simulink model "optimized_area_multi_module_phase_shift_generator_built_in_counter"  (R2025b)
settings: Solver=FixedStepDiscrete  StartTime=0.0  StopTime=10e3  RelTol=1e-3
libraries: hdlsllib x1
settings Model: DataTypeOverride=Off  FPTShortcutValueString='{{},{''BaselineRun'',1,1,1,''BaselineRun'','''',{},''M'',''F'',''''}}'  Creator=KoayXianCong  LastModifiedBy=KoayXianCong
settings OptimizationCC: BlockReduction=off  ConditionallyExecuteInputs=off  DefaultParameterBehavior=Inlined  InheritOutputTypeSmallerThanSingle=on
settings DebuggingCC: SignalRangeChecking=warning  ArtificialAlgebraicLoopMsg=error  SingleTaskRateTransMsg=error
settings HardwareCC: ProdBitPerPointer=32.0  ProdBitPerSizeT=32.0  ProdBitPerPtrDiffT=32.0  ProdLargestAtomicFloat=None  ProdIntDivRoundTo=Undefined  ProdEndianess=Unspecified  ProdWordSize=32.0  ProdHWDeviceType=ASIC/FPGA->ASIC/FPGA  TargetBitPerPointer=64.0  TargetBitPerSizeT=64.0  TargetBitPerPtrDiffT=64.0  TargetLongLongMode=on  TargetIntDivRoundTo=Zero  TargetEndianess=LittleEndian  TargetWordSize=64.0  TargetHWDeviceType=Custom Processor->MATLAB Host Computer  ProdEqTarget=off

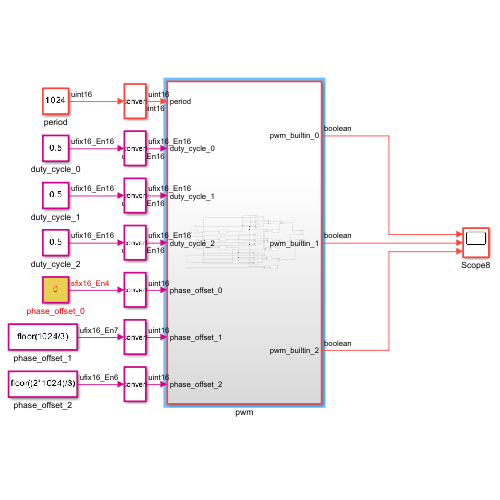
[thumbnail: Simulink's stored preview of the top-level diagram]
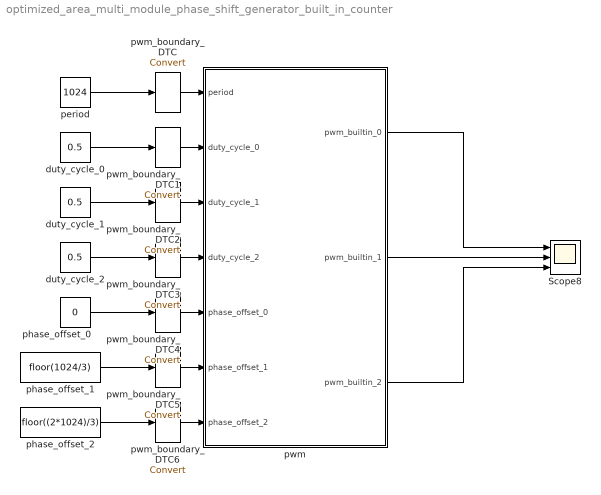
== system optimized_area_multi_module_phase_shift_generator_built_in_counter ==
  Scope8 : Scope  NumInputPorts=3
      settings: ActiveDisplayYMinimum=-1  ActiveDisplayYMaximum=1  DataLoggingVariableName=ScopeData10  DataLoggingSaveFormat=Array
  duty_cycle_0 : Constant  Value=0.5  OutDataTypeStr=fixdt(0,16,16)
  duty_cycle_1 : Constant  Value=0.5  OutDataTypeStr=fixdt(0,16,16)
  duty_cycle_2 : Constant  Value=0.5  OutDataTypeStr=fixdt(0,16,16)
  period : Constant  Value=1024  OutDataTypeStr=uint16  SampleTime=1
  phase_offset_0 : Constant  Value=0  OutDataTypeStr=fixdt(1,16,4)
  phase_offset_1 : Constant  Value=floor(1024/3)  OutDataTypeStr=fixdt(0,16,7)
  phase_offset_2 : Constant  Value=floor((2*1024)/3)  OutDataTypeStr=fixdt(0,16,6)
  pwm : Subsystem
  pwm_boundary_DTC{,1..6} (7 alike) : DataTypeConversion
  wires:
  pwm/1(pwm_builtin_0) -> Scope8/1
  pwm/2(pwm_builtin_1) -> Scope8/2
  pwm/3(pwm_builtin_2) -> Scope8/3
  period/1 -> pwm_boundary_DTC/1
  pwm_boundary_DTC/1 -> pwm/1(period)
  duty_cycle_0/1 -> pwm_boundary_DTC1/1
  pwm_boundary_DTC1/1 -> pwm/2(duty_cycle_0)
  duty_cycle_1/1 -> pwm_boundary_DTC2/1
  pwm_boundary_DTC2/1 -> pwm/3(duty_cycle_1)
  duty_cycle_2/1 -> pwm_boundary_DTC3/1
  pwm_boundary_DTC3/1 -> pwm/4(duty_cycle_2)
  phase_offset_0/1 -> pwm_boundary_DTC4/1
  pwm_boundary_DTC4/1 -> pwm/5(phase_offset_0)
  phase_offset_1/1 -> pwm_boundary_DTC5/1
  pwm_boundary_DTC5/1 -> pwm/6(phase_offset_1)
  phase_offset_2/1 -> pwm_boundary_DTC6/1
  pwm_boundary_DTC6/1 -> pwm/7(phase_offset_2)

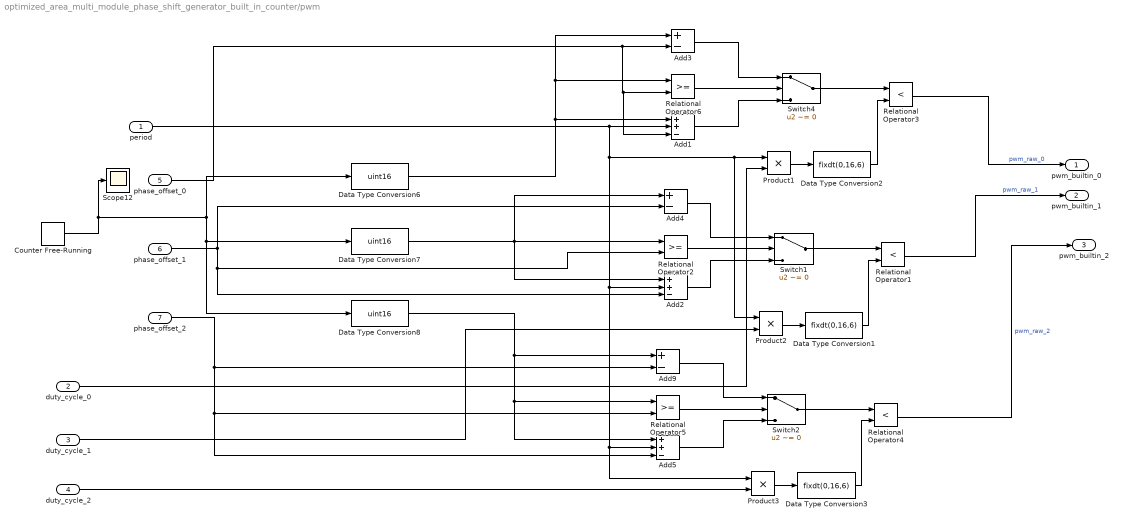
== system optimized_area_multi_module_phase_shift_generator_built_in_counter/pwm ==
  period : Inport  OutDataTypeStr=uint16
  duty_cycle_0 : Inport  Port=2  OutDataTypeStr=fixdt(0,16,16)
  duty_cycle_1 : Inport  Port=3  OutDataTypeStr=fixdt(0,16,16)
  duty_cycle_2 : Inport  Port=4  OutDataTypeStr=fixdt(0,16,16)
  phase_offset_0 : Inport  Port=5
  phase_offset_1 : Inport  Port=6
  phase_offset_2 : Inport  Port=7
  Add1 : Sum  Inputs=++-
  Add2 : Sum  Inputs=++-
  Add3 : Sum  Inputs=+-
  Add4 : Sum  Inputs=+-
  Add5 : Sum  Inputs=++-
  Add9 : Sum  Inputs=+-
  Counter Free-Running : hdlsllib/Sources/Counter Free-Running  NumBits=10  tsamp=1
  Data Type Conversion1 : DataTypeConversion  OutDataTypeStr=fixdt(0,16,6)  SaturateOnIntegerOverflow=off  RndMeth=Floor
  Data Type Conversion2 : DataTypeConversion  OutDataTypeStr=fixdt(0,16,6)  SaturateOnIntegerOverflow=off  RndMeth=Floor
  Data Type Conversion3 : DataTypeConversion  OutDataTypeStr=fixdt(0,16,6)  SaturateOnIntegerOverflow=off  RndMeth=Floor
  Data Type Conversion6 : DataTypeConversion  OutDataTypeStr=uint16  SaturateOnIntegerOverflow=off  RndMeth=Floor
  Data Type Conversion7 : DataTypeConversion  OutDataTypeStr=uint16  SaturateOnIntegerOverflow=off  RndMeth=Floor
  Data Type Conversion8 : DataTypeConversion  OutDataTypeStr=uint16  SaturateOnIntegerOverflow=off  RndMeth=Floor
  Product1 : Product  OutDataTypeStr=fixdt(0,16,6)
  Product2 : Product  OutDataTypeStr=fixdt(0,16,6)
  Product3 : Product  OutDataTypeStr=fixdt(0,16,6)
  Relational Operator1 : RelationalOperator  Operator=<  OutDataTypeStr=boolean  RndMeth=Simplest  InputSameDT=off
  Relational Operator2 : RelationalOperator  OutDataTypeStr=boolean  InputSameDT=off
  Relational Operator3 : RelationalOperator  Operator=<  OutDataTypeStr=boolean  RndMeth=Simplest  InputSameDT=off
  Relational Operator4 : RelationalOperator  Operator=<  OutDataTypeStr=boolean  RndMeth=Simplest  InputSameDT=off
  Relational Operator5 : RelationalOperator  OutDataTypeStr=boolean  InputSameDT=off
  Relational Operator6 : RelationalOperator  OutDataTypeStr=boolean  InputSameDT=off
  Scope12 : Scope
      settings: ActiveDisplayYMinimum=-127.87499999999997  ActiveDisplayYMaximum=1150.875  DataLoggingVariableName=ScopeData12  DataLoggingSaveFormat=Array
  Switch1 : Switch  Criteria=u2 ~= 0  SaturateOnIntegerOverflow=off  InputSameDT=off
  Switch2 : Switch  Criteria=u2 ~= 0  SaturateOnIntegerOverflow=off  InputSameDT=off
  Switch4 : Switch  Criteria=u2 ~= 0  SaturateOnIntegerOverflow=off  InputSameDT=off
  pwm_builtin_0 : Outport
  pwm_builtin_1 : Outport  Port=2
  pwm_builtin_2 : Outport  Port=3
  wires:
  phase_offset_1/1 -> Add4/2, Add2/3, Relational Operator2/2
  phase_offset_2/1 -> Add5/3, Relational Operator5/2, Add9/2
  Counter Free-Running/1 -> Scope12/1, Data Type Conversion8/1, Data Type Conversion7/1, Data Type Conversion6/1
  phase_offset_0/1 -> Add1/3, Relational Operator6/2, Add3/2
  Data Type Conversion6/1 -> Relational Operator6/1, Add3/1, Add1/1
  period/1 -> Product3/1, Add5/2, Add2/2, Product2/1, Product1/1, Add1/2
  Add3/1 -> Switch4/1
  Relational Operator6/1 -> Switch4/2
  Add1/1 -> Switch4/3
  Switch4/1 -> Relational Operator3/1
  Product1/1 -> Data Type Conversion2/1
  Data Type Conversion2/1 -> Relational Operator3/2
  Relational Operator3/1 -> pwm_builtin_0/1  "pwm_raw_0"
  Data Type Conversion7/1 -> Add2/1, Relational Operator2/1, Add4/1
  Product2/1 -> Data Type Conversion1/1
  Data Type Conversion1/1 -> Relational Operator1/2
  Switch1/1 -> Relational Operator1/1
  Add4/1 -> Switch1/1
  Relational Operator2/1 -> Switch1/2
  Add2/1 -> Switch1/3
  Relational Operator1/1 -> pwm_builtin_1/1  "pwm_raw_1"
  Data Type Conversion8/1 -> Add5/1, Relational Operator5/1, Add9/1
  Product3/1 -> Data Type Conversion3/1
  Data Type Conversion3/1 -> Relational Operator4/2
  Switch2/1 -> Relational Operator4/1
  Add9/1 -> Switch2/1
  Relational Operator5/1 -> Switch2/2
  Add5/1 -> Switch2/3
  Relational Operator4/1 -> pwm_builtin_2/1  "pwm_raw_2"
  duty_cycle_0/1 -> Product1/2
  duty_cycle_1/1 -> Product2/2
  duty_cycle_2/1 -> Product3/2
